simulink model "child2_mulbox"  (R2013b)
settings: Solver=ode3  SolverMode=SingleTasking  StartTime=0.0  StopTime=10.0  RelTol=1e-3
libraries: legonxtlib x6, simulink x1
settings Model: ExtModeTrigDuration=2  Creator=grouleau  LastModifiedBy=mouyang
settings DataIOCC: SignalLoggingSaveFormat=ModelDataLogs
settings OptimizationCC: OptimizeModelRefInitCode=on  LifeSpan=1
settings DebuggingCC: SolverPrmCheckMsg=none  MultiTaskDSMMsg=warning  MultiTaskCondExecSysMsg=none
settings HardwareCC: ProdLargestAtomicInteger=Long  ProdLargestAtomicFloat=Float  ProdEndianess=LittleEndian  ProdHWDeviceType=ARM Compatible->ARM 7
settings RTWCC: SystemTargetFile=realtime.tlc  GenerateMakefile=off  TemplateMakefile=realtime.tmf  Description=Run on Target Hardware  RTWVerbose=off  ProcessScript=realtime_make_rtw_hook  IncludeERTFirstTime=on
settings STFCustomTargetCC: TargetLibSuffix=.a  GenerateSampleERTMain=on  ERTCustomFileBanners=on  SupportNonInlinedSFcns=off  SupportVariableSizeSignals=on  MATLABClassNameForMDSCustomization=Simulink.SoftwareTarget.ERTCustomization  GRTInterface=off  SystemTargetFile=realtime.tlc
settings ERTTargetCC: CodeReplacementLibrary=ANSI_C  GenerateSampleERTMain=on  ParMdlRefBuildCompliant=off  CompOptLevelCompliant=off  ConcurrentExecutionCompliant=off  CombineOutputUpdateFcns=off  ERTFirstTimeCompliant=off  SupportContinuousTime=on  SupportVariableSizeSignals=on  ModelStepFunctionPrototypeControlCompliant=off  CPPClassGenCompliant=off  ExtModeTransport=1  ExtModeMexFile=ext_serial_win32_comm_no_acks_rtt_byteswap  ExtModeMexArgs=0 1 9600  InlinedParameterPlacement=NonHierarchical  ERTSrcFileBannerTemplate=realtime_code_template.cgt  ERTHdrFileBannerTemplate=realtime_code_template.cgt  ERTDataSrcFileTemplate=realtime_code_template.cgt  ERTDataHdrFileTemplate=realtime_code_template.cgt  ERTCustomFileTemplate=realtime_file_process.tlc

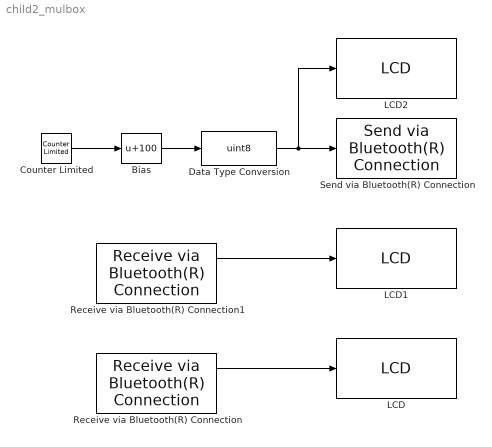
== system child2_mulbox ==
  Bias : Bias  Bias=100
  Counter Limited : simulink/Sources/Counter Limited  uplimit=7  tsamp=1
  Data Type Conversion : DataTypeConversion  OutDataTypeStr=uint8
  LCD : legonxtlib/LCD  slcdStr=MB3  slcdLine=1  slcdFormat=Decimal
  LCD1 : legonxtlib/LCD  slcdStr=MB5  slcdLine=2  slcdFormat=Decimal
  LCD2 : legonxtlib/LCD  slcdStr=MB4  slcdLine=3  slcdFormat=Decimal
  Receive via Bluetooth(R) Connection : legonxtlib/Receive via Bluetooth(R) Connection  mailbox=3  dataType=uint8  dataSize=1  sampleTime=1
  Receive via Bluetooth(R) Connection1 : legonxtlib/Receive via Bluetooth(R) Connection  mailbox=5  dataType=uint8  dataSize=1  sampleTime=1
  Send via Bluetooth(R) Connection : legonxtlib/Send via Bluetooth(R) Connection  mailbox=4
  wires:
  Counter Limited/1 -> Bias/1
  Data Type Conversion/1 -> LCD2/1, Send via Bluetooth(R) Connection/1
  Bias/1 -> Data Type Conversion/1
  Receive via Bluetooth(R) Connection/1 -> LCD/1
  Receive via Bluetooth(R) Connection1/1 -> LCD1/1
